simulink subsystem "Vehicle1D_refsub_Custom"  (R2022a)
settings: Solver=VariableStepAuto  StartTime=0.0  StopTime=10.0  RelTol=1e-3
libraries: nesl_utility x8, fl_lib x4
settings Model: Creator=isaacito  LastModifiedBy=isaacito
settings SolverCC: AlgebraicLoopSolver=TrustRegion
settings DebuggingCC: UnconnectedInputMsg=warning  UnconnectedOutputMsg=warning  UnconnectedLineMsg=warning  SFMachineParentedDataDiag=warning
settings RTWCC: DLArmComputeVersion=19.05

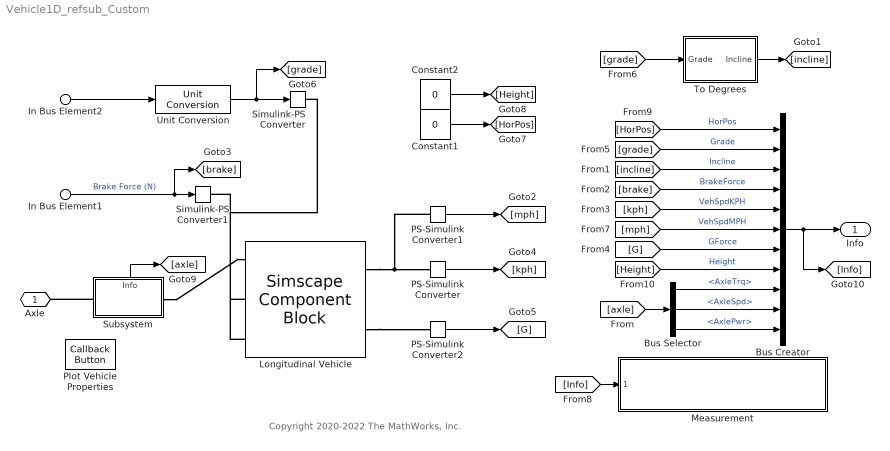
== system Vehicle1D_refsub_Custom ==
  note: Copyright 2020-2022 The MathWorks, Inc.
  In Bus Element1 : Inport  PortName=Inputs  Element=BrakeForce
      settings: AttributesFormatString=%<Unit>
  In Bus Element2 : Inport  PortName=Inputs  Element=RoadGrade
      settings: AttributesFormatString=%<Unit>
  Bus Creator : BusCreator  Inputs=11
  Bus Selector : BusSelector  OutputSignals=AxleTrq,AxleSpd,AxlePwr
  Constant1 : Constant  Value=0
  Constant2 : Constant  Value=0
  Longitudinal Vehicle : SimscapeComponentBlock  SourceFile=Vehicle1D_Custom  ComponentPath=Vehicle1D_Custom  ComponentVariants="[\"Vehicle1D_Custom\"]"  ComponentVariantNames="[\"Vehicle1D_Custom\"]"  ClassName=Vehicle1D_Custom  SchemaVersion=1  grav=vehicle.roadLoad_gravAccel_m_per_s2 m/s^2  M_e=vehicle.mass_kg kg  R_tire=vehicle.tireRollingRadius_m m  A_rl=vehicle.roadLoadA_N N  B_rl=vehicle.roadLoadB_N_per_kph N*hr/km  C_rl=vehicle.roadLoadC_N_per_kph2 N*hr^2/km^2  V_1=smoothing.vehicle_speedThreshold_kph km/hr  w_1=smoothing.vehicle_axleSpeedThreshold_rpm rpm  V_x_specify=on  V_x_priority=High  V_x=initial.vehicle_speed_kph km/hr  V_x_nominal_specify=off  V_x_nominal_unit=km/hr  V_x_nominal_value=1
      settings: AttributesFormatString=%<V_x>  CopyFcn=simscape.engine.sli.internal.componentblockcallback(gcbh,'COPY')  PreCopyFcn=simscape.engine.sli.internal.componentblockcallback(gcbh,'PRECOPY')  PreDeleteFcn=simscape.engine.sli.internal.componentblockcallback(gcbh,'PREDELETE')  LogSimulationData=on  InternalSimscapePortConfiguration="{\"Bottom\":[],\"Left\":[{\"id\":\"Axle\",\"label\":\"Axle\",\"type\":\"foundation.mechanical.rotational.rotational\"}],\"Right\":[{\"id\":\"v_out\",\"label\":\"V\",\"type\":\"output\"},{\"id\":\"G\",\"label\":\"G\",\"type\":\"output\"}],\"Top\":[{\"id\":\"brkF\",\"label\":\"Brake\",\"type\":\"input\"},{\"id\":\"grade_norm\",\"label\":\"Grade\",\"type\":\"input\"}]}"
      mask Type: Custom Longitudinal Vehicle
  Measurement : Subsystem  ReferencedSubsystem=Vehicle1D_measurement_refsub_logging
  PS-Simulink Converter : nesl_utility/PS-Simulink Converter  PhysicalDomain=network_engine_domain  SubClassName=ps_output  LeftPortType=input  RightPortType=output  PseudoPeriodic=off  Frequencies=[]  VectorFormat=1-D array  Unit=km/hr  AffineConversion=off
      settings: SourceProductBaseCode=SS,PW,VE
  PS-Simulink Converter1 : nesl_utility/PS-Simulink Converter  PhysicalDomain=network_engine_domain  SubClassName=ps_output  LeftPortType=input  RightPortType=output  PseudoPeriodic=off  Frequencies=[]  VectorFormat=1-D array  Unit=mph  AffineConversion=off
      settings: SourceProductBaseCode=SS,PW,VE
  PS-Simulink Converter2 : nesl_utility/PS-Simulink Converter  PhysicalDomain=network_engine_domain  SubClassName=ps_output  LeftPortType=input  RightPortType=output  PseudoPeriodic=off  Frequencies=[]  VectorFormat=1-D array  Unit=1  AffineConversion=off
      settings: SourceProductBaseCode=SS,PW,VE
  Plot Vehicle Properties : CallbackButton  ButtonText=Plot
      settings: ClickFcn=|
      | % Select the block.
      | set_param(gcs, CurrentBlock="Longitudinal Vehicle")
      | 
      | Vehicle1D_plotProperties_Custom(gcbh);
  Simulink-PS Converter : nesl_utility/Simulink-PS Converter  PhysicalDomain=network_engine_domain  SubClassName=ps_input  LeftPortType=input  RightPortType=output  PseudoPeriodic=off  Frequencies=[]  NoiseDistribution=none  NoiseParameters=[]  Unit=1  AffineConversion=off  FilteringAndDerivatives=filter  SimscapeFilterOrder=1  InputFilterTimeConstant=0.001  UdotUserProvided=0
      settings: SourceProductBaseCode=SS,PW,VE
  Simulink-PS Converter1 : nesl_utility/Simulink-PS Converter  PhysicalDomain=network_engine_domain  SubClassName=ps_input  LeftPortType=input  RightPortType=output  PseudoPeriodic=off  Frequencies=[]  NoiseDistribution=none  NoiseParameters=[]  Unit=N  AffineConversion=off  FilteringAndDerivatives=filter  SimscapeFilterOrder=1  InputFilterTimeConstant=0.001  UdotUserProvided=0
      settings: SourceProductBaseCode=SS,PW,VE
  Subsystem : Subsystem
      settings: PortSchema="{\"entries\":[{\"content\":{\"sides\":[{\"content\":{\"connectorIds\":[\"LConn1\"]},\"type\":\"ConnectorPlacement.EquallySpacedRectSide\",\"uuid\":\"ec3cd8f6-c333-4ae9-94e8-194dcd7a9a9d\"},{\"content\":{\"connectorIds\":[\"RConn1\"],\"side\":\"RIGHT\"},\"type\":\"ConnectorPlacement.EquallySpacedRectSide\",\"uuid\":\"fef4b050-361f-4de4-b245-db8f722dbe30\"},{\"content\":{\"connectorIds\":[\"Out1\"],\"side\":\"TOP\"},\"type\":\"ConnectorPlacement.EquallySpacedRectSide\",\"uuid\":\"eda11c3e-d822-4525-9660-298bf232b628\"}]},\"type\":\"ConnectorPlacement.EquallySpacedConnector\",\"uuid\":\"afcb7fc3-0a34-49fa-b864-b9b6e2272b9d\"}],\"packageUris\":[\"http://schema.mathworks.com/mf0/Connector/R2020b\"],\"version\":\"1.0\"}"
  To Degrees : Subsystem
  Unit Conversion : UnitConversion
  Axle : PMIOPort  Side=Left
  Info : Outport
  wires:
  PS-Simulink Converter/1 -> [kph]
  PS-Simulink Converter2/1 -> [G]
  In Bus Element1/1 -> [brake], Simulink-PS Converter1/1  "Brake Force (N)"
  Subsystem/1(Info) -> [axle]
  [grade] -> To Degrees/1(Grade)
  To Degrees/1(Incline) -> [incline]
  PS-Simulink Converter1/1 -> [mph]
  Constant1/1 -> [HorPos]
  Constant2/1 -> [Height]
  Bus Selector/3 -> Bus Creator/11  "<AxlePwr>"
  Bus Selector/1 -> Bus Creator/9  "<AxleTrq>"
  Bus Selector/2 -> Bus Creator/10  "<AxleSpd>"
  [Height] -> Bus Creator/8  "Height"
  [mph] -> Bus Creator/6  "VehSpdMPH"
  [HorPos] -> Bus Creator/1  "HorPos"
  [kph] -> Bus Creator/5  "VehSpdKPH"
  Bus Creator/1 -> Info/1, [Info]
  [grade] -> Bus Creator/2  "Grade"
  [Info] -> Measurement/1
  [axle] -> Bus Selector/1
  [brake] -> Bus Creator/4  "BrakeForce"
  [incline] -> Bus Creator/3  "Incline"
  [G] -> Bus Creator/7  "GForce"
  Unit Conversion/1 -> Simulink-PS Converter/1, [grade]
  In Bus Element2/1 -> Unit Conversion/1
  connections:
  PS-Simulink Converter1/LConn1 -- Longitudinal Vehicle/RConn1 -- PS-Simulink Converter/LConn1
  Longitudinal Vehicle/RConn2 -- PS-Simulink Converter2/LConn1
  Longitudinal Vehicle/LConn3 -- Simulink-PS Converter/RConn1
  Longitudinal Vehicle/LConn2 -- Simulink-PS Converter1/RConn1
  Subsystem/RConn1 -- Longitudinal Vehicle/LConn1
  Subsystem/LConn1 -- Axle/RConn1

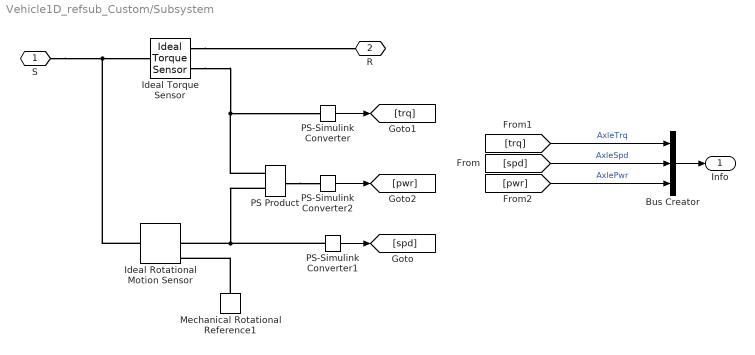
== system Vehicle1D_refsub_Custom/Subsystem ==
  Bus Creator : BusCreator  Inputs=3
  Ideal Rotational Motion Sensor : fl_lib/Mechanical/Mechanical Sensors/Ideal Rotational Motion Sensor  wrap_angle=simscape.enum.onoff.off  offset=0 rad
      settings: SourceProductBaseCode=PW,SS,VE
  Ideal Torque Sensor : fl_lib/Mechanical/Mechanical Sensors/Ideal Torque Sensor
      settings: SourceProductBaseCode=PW,SS,VE
  Mechanical Rotational Reference1 : fl_lib/Mechanical/Rotational Elements/Mechanical Rotational Reference
      settings: SourceProductBaseCode=PW,SS,VE
  PS Product : fl_lib/Physical Signals/Functions/PS Product
      settings: SourceProductBaseCode=PW,SS,VE
  PS-Simulink Converter : nesl_utility/PS-Simulink Converter  PhysicalDomain=network_engine_domain  SubClassName=ps_output  LeftPortType=input  RightPortType=output  PseudoPeriodic=off  Frequencies=[]  VectorFormat=inherit  Unit=N*m  AffineConversion=off
      settings: SourceProductBaseCode=SS,PW,VE
  PS-Simulink Converter1 : nesl_utility/PS-Simulink Converter  PhysicalDomain=network_engine_domain  SubClassName=ps_output  LeftPortType=input  RightPortType=output  PseudoPeriodic=off  Frequencies=[]  VectorFormat=1-D array  Unit=rpm  AffineConversion=off
      settings: SourceProductBaseCode=SS,PW,VE
  PS-Simulink Converter2 : nesl_utility/PS-Simulink Converter  PhysicalDomain=network_engine_domain  SubClassName=ps_output  LeftPortType=input  RightPortType=output  PseudoPeriodic=off  Frequencies=[]  VectorFormat=inherit  Unit=kW  AffineConversion=off
      settings: SourceProductBaseCode=SS,PW,VE
  S : PMIOPort  Side=Left
  R : PMIOPort  Port=2  Side=Right
  Info : Outport
  wires:
  Bus Creator/1 -> Info/1
  [pwr] -> Bus Creator/3  "AxlePwr"
  [spd] -> Bus Creator/2  "AxleSpd"
  [trq] -> Bus Creator/1  "AxleTrq"
  PS-Simulink Converter2/1 -> [pwr]
  PS-Simulink Converter/1 -> [trq]
  PS-Simulink Converter1/1 -> [spd]
  connections:
  PS Product/RConn1 -- PS-Simulink Converter2/LConn1
  PS Product/LConn1 -- PS-Simulink Converter/LConn1 -- Ideal Torque Sensor/RConn2
  Ideal Torque Sensor/RConn1 -- R/RConn1
  Ideal Rotational Motion Sensor/LConn1 -- S/RConn1 -- Ideal Torque Sensor/LConn1
  PS Product/LConn2 -- PS-Simulink Converter1/LConn1 -- Ideal Rotational Motion Sensor/RConn2
  Mechanical Rotational Reference1/LConn1 -- Ideal Rotational Motion Sensor/RConn1

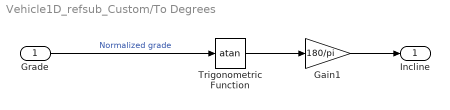
== system Vehicle1D_refsub_Custom/To Degrees ==
  Grade : Inport  Unit=1
      settings: AttributesFormatString=%<Unit>
  Gain1 : Gain  Gain=180/pi
  Trigonometric Function : Trigonometry  Operator=atan
  Incline : Outport  Unit=deg
      settings: AttributesFormatString=%<Unit>
  wires:
  Grade/1 -> Trigonometric Function/1  "Normalized grade"
  Trigonometric Function/1 -> Gain1/1
  Gain1/1 -> Incline/1
